simulink model "FOTON_BMS_DEM"  (Simulink 7.4)
settings: Solver=FixedStepDiscrete  StartTime=0.0  StopTime=inf  FixedStep=BMS_Const_TickTm_s  RelTol=1e-3
CloseFcn:
  | rtwprivate ssgencode ModelCloseRequest FOTON_BMS_STRATEGY
settings Model: Creator=zhaoxiangri  LastModifiedBy=sunsijun
settings DataIOCC: SaveFormat=StructureWithTime  SaveOutput=off  SaveTime=off
settings OptimizationCC: InlineParams=on  InlineInvariantSignals=on  ExpressionDepthLimit=128  StateBitsets=on  DataBitsets=on  UseTempVars=on  ZeroExternalMemoryAtStartup=off  ZeroInternalMemoryAtStartup=off  NoFixptDivByZeroProtection=on  EfficientFloat2IntCast=on  OptimizeModelRefInitCode=on  LifeSpan=Inf
settings DebuggingCC: RTPrefix=none  SignalInfNanChecking=warning  CheckSSInitialOutputMsg=off  SignalResolutionControl=TryResolveAll  MultiTaskCondExecSysMsg=warning  MultiTaskRateTransMsg=warning  IntegerOverflowMsg=error  ParameterDowncastMsg=none  ParameterPrecisionLossMsg=none  UnnecessaryDatatypeConvMsg=warning  FcnCallInpInsideContextMsg=Enable All  UnconnectedInputMsg=error  UnconnectedOutputMsg=error  UnconnectedLineMsg=error  UniqueDataStoreMsg=error  RootOutportRequireBusObject=none  ModelReferenceIOMsg=warning  ModelReferenceVersionMismatchMessage=warning  ModelReferenceIOMismatchMessage=warning  ModelReferenceCSMismatchMessage=warning  StrictBusMsg=ErrorLevel1
settings HardwareCC: ProdIntDivRoundTo=Zero  ProdEndianess=BigEndian  ProdHWDeviceType=Freescale->32-bit PowerPC
settings RTWCC: SystemTargetFile=ert.tlc  GenCodeOnly=on  TemplateMakefile=ert_default_tmf  Description=Real-Time Workshop Embedded Coder  GenerateReport=on  RTWVerbose=off  ProcessScript=ert_make_rtw_hook  IncludeHyperlinkInReport=on  LaunchReport=on  GenerateTraceInfo=on  GenerateTraceReport=on  GenerateTraceReportSl=on  GenerateTraceReportSf=on  GenerateTraceReportEml=on
settings CodeAppCC: ForceParamTrailComments=on  IgnoreCustomStorageClasses=off  SimulinkDataObjDesc=on  CustomSymbolStrGlobalVar=rt$N$M  CustomSymbolStrType=$N$M  CustomSymbolStrFcn=$N$M$F  CustomSymbolStrMacro=$N$M  InsertBlockDesc=on
settings ERTTargetCC: MultiwordLength=2048  GenerateASAP2=on  InlinedParameterPlacement=NonHierarchical  ERTCustomFileTemplate=example_file_process.tlc  GlobalDataDefinition=InSeparateSourceFile  DataDefinitionFile=var.c  GlobalDataReference=InSeparateHeaderFile  DataReferenceFile=var.h  ConvertIfToSwitch=off

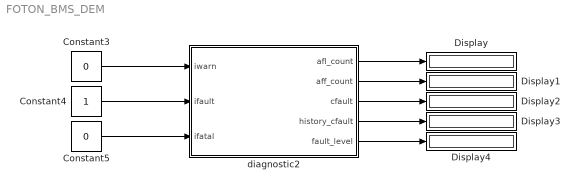
== system FOTON_BMS_DEM ==
  Constant3 : Constant  Value=0  OutDataTypeMode=boolean  OutDataType=fixdt(1, 16)  OutScaling=2^0  OutDataTypeStr=boolean
  Constant4 : Constant  OutDataTypeMode=boolean  OutDataType=fixdt(1, 16)  OutScaling=2^0  OutDataTypeStr=boolean
  Constant5 : Constant  Value=0  OutDataTypeMode=boolean  OutDataType=fixdt(1, 16)  OutScaling=2^0  OutDataTypeStr=boolean
  Display{,1..4} (5 alike) : Display
  diagnostic2 : Subsystem  TreatAsAtomicUnit=on  RTWFcnName=diagnostic  mask(Fault_Diagnostic){afl_inc=3, afl_dec=3, afl_threshold=10, aff_threshold=255}
      mask prompts: afl_inc "AFL_INCREMENT"; afl_dec "AFL_DECREMENT"
      mask help:
      | AFL:Accumulated Failure Level.
      | AFF:Accumulated Failure Frequency
      | AFL_INCREMENT:The value of the internal counter gets incremented each cycle if the ifault is active [uint8] [0...255].
      | AFL_DECREMENT:The value of  the internal counter gets decremented each cycle if the ifault is inactive [uint8] [0...255].
      | AFL_THRESHOLD:When the internal counter is more than AFL_THRESHOLD,fault is confirmed.
      | AFF_THRESHOLD:The aff_count must be less than AFF_THRESHOLD.
      settings: AttributesFormatString=[AFL_INCREMENT=%<afl_inc>]\n[AFL_DECREMENT=%<afl_dec>]\n[AFL_THRESHOLD=%<afl_threshold>]\n[AFF_THRESHOLD=%<aff_threshold>]  RTWFcnNameOpts=User specified
      mask Display:
      | disp('DIAGNOSTIC')
      | port_label('input',1,'iwarn')
      | port_label('input',2,'ifault')
      | port_label('input',3,'ifatal')
      | port_label('output',1,'afl_count')
      | port_label('output',2,'aff_count')
      | port_label('output',3,'cfault')
      | port_label('output',4,'history_cfault')
      | port_label('output',5,'fault_level')
  wires:
  Constant3/1 -> diagnostic2/1(iwarn)
  Constant4/1 -> diagnostic2/2(ifault)
  Constant5/1 -> diagnostic2/3(ifatal)
  diagnostic2/1(afl_count) -> Display/1
  diagnostic2/5(fault_level) -> Display4/1
  diagnostic2/2(aff_count) -> Display1/1
  diagnostic2/3(cfault) -> Display2/1
  diagnostic2/4(history_cfault) -> Display3/1

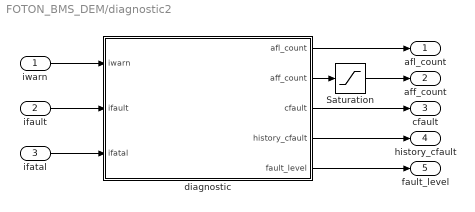
== system FOTON_BMS_DEM/diagnostic2 ==
  iwarn : Inport  OutDataType=fixdt(1, 16)  OutScaling=2^0
  ifault : Inport  Port=2  OutDataType=fixdt(1, 16)  OutScaling=2^0
  ifatal : Inport  Port=3  OutDataType=fixdt(1, 16)  OutScaling=2^0
  Saturation : Saturate  UpperLimit=aff_threshold  LowerLimit=0  OutDataType=fixdt(1, 16)  OutScaling=2^0
  diagnostic : Stateflow chart  TreatAsAtomicUnit=on
  afl_count : Outport
  aff_count : Outport  Port=2
  cfault : Outport  Port=3
  history_cfault : Outport  Port=4
  fault_level : Outport  Port=5
  wires:
  diagnostic/5(fault_level) -> fault_level/1
  ifatal/1 -> diagnostic/3(ifatal)
  iwarn/1 -> diagnostic/1(iwarn)
  ifault/1 -> diagnostic/2(ifault)
  diagnostic/1(afl_count) -> afl_count/1
  diagnostic/3(cfault) -> cfault/1
  diagnostic/4(history_cfault) -> history_cfault/1
  diagnostic/2(aff_count) -> Saturation/1
  Saturation/1 -> aff_count/1

== stateflow chart diagnostic2/diagnostic ==
  state Fault_Diagnostic
    state No_Cfault
      cfault=0;
      counter=0;
      fault_level=0;
      afl_count=counter;
    state Counter
      state AFL_DEC
        (junction 11) -> (junction 12) : {afl_count=counter;counter-=afl_dec;}
        (default) -> (junction 11)
        AFL_DEC -> (junction 11) [order 1]
      state AFL_INC
        (default) -> (junction 9)
        (junction 9) -> (junction 10) : {afl_count=counter;counter+=afl_inc;}
        AFL_INC -> (junction 9) [order 1]
      AFL_INC -> AFL_DEC [order 2] : [iwarn==0&&...
          | ifault==0&&...
          | ifatal==0&&...
          | counter<afl_threshold]
      AFL_DEC -> AFL_INC [order 2] : [(iwarn==1||...
          | ifault==1||...
          | ifatal==1)&&...
          | counter>0]
    state Cfault
      (default) -> (junction 15) : {afl_count=afl_threshold;
          | counter=afl_threshold;
          | cfault=1;
          | history_cfault=1;
          | aff_count++;}
      (junction 22) -> (junction 21)
      (junction 15) -> (junction 16) [order 1] : [iwarn==1]
      (junction 16) -> (junction 18) : {fault_level = 1;}
      (junction 15) -> (junction 18) [order 2]
      (junction 18) -> (junction 17) [order 1] : [ifault==1]
      (junction 17) -> (junction 20) : {fault_level = 2;}
      (junction 18) -> (junction 20) [order 2]
      (junction 20) -> (junction 19) [order 1] : [ifatal==1]
      (junction 19) -> (junction 22) : {fault_level = 3;}
      (junction 20) -> (junction 22) [order 2]
    (default) -> No_Cfault : {aff_count=0;}
    No_Cfault -> AFL_INC : [iwarn==1||...
        | ifault==1||...
        | ifatal==1]
    AFL_DEC -> (junction 14) [order 1] : [counter<=0]
    AFL_INC -> (junction 13) [order 1] : [counter>=afl_threshold]
    Cfault -> AFL_DEC : [iwarn==0&&...
        | ifault==0&&...
        | ifatal==0]
    (junction 13) -> Cfault
    (junction 14) -> No_Cfault
  (default) -> Fault_Diagnostic
  data: iwarn input boolean; afl_count output int16; aff_count output uint8; afl_dec parameter uint8; afl_inc parameter uint8; afl_threshold parameter uint8; cfault output boolean; history_cfault output boolean; ifault input boolean; aff_threshold parameter uint8; counter local int16; ifatal input boolean; fault_level output uint8
